simulink library "Weather_Datafile"  (R2018b)
settings: Solver=ode45  StartTime=0.0  StopTime=10.0  RelTol=1e-3  EnableMultiTasking=on
undefined symbols (not defined in the file): DE_TRY2010_04_averageYear, path_carnot
libraries: carnot x1
settings Model: Creator=Bernd.Hafner  LastModifiedBy=P41573
settings DataIOCC: LimitDataPoints=on  SaveFormat=Array  SignalLoggingSaveFormat=ModelDataLogs
settings OptimizationCC: ExpressionDepthLimit=2147483647  LifeSpan=inf
settings DebuggingCC: UnderspecifiedInitializationDetection=Classic  MergeDetectMultiDrivingBlocksExec=none  SolverPrmCheckMsg=warning  FcnCallInpInsideContextMsg=warning  StateNameClashWarn=warning  SFUnexpectedBacktrackingDiag=warning  SFNoUnconditionalDefaultTransitionDiag=warning  SFExecutionAtInitializationDiag=none
settings HardwareCC: ProdBitPerPointer=32  ProdBitPerSizeT=32  ProdBitPerPtrDiffT=32  ProdLargestAtomicFloat=None  ProdIntDivRoundTo=Undefined  ProdEndianess=Unspecified  ProdWordSize=32  ProdHWDeviceType=32-bit Generic
settings ModelReferenceCC: PropagateSignalLabelsOutOfModel=off
settings SFSimCC: SimUseLocalCustomCode=off
settings RTWCC: RTWUseLocalCustomCode=off
settings CodeAppCC: StateflowObjectComments=on
settings GRTTargetCC: TargetLangStandard=C89/C90 (ANSI)  GeneratePreprocessorConditionals=Disable all  CombineOutputUpdateFcns=off  GRTInterface=on
settings ConfigComp: CovMetricSettings=dw  CovHtmlReporting=on  CovSaveCumulativeToWorkspaceVar=on  CovSaveSingleToWorkspaceVar=on  CovExternalEMLEnable=off

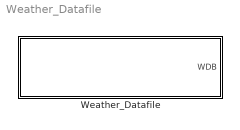
== system Weather_Datafile ==
  Weather_Datafile : Subsystem  mask(Weather Datafile){PathName=path_carnot('data'), FileName='DE_TRY2010_04_averageYear.mat', UserParam=off, VariableName=DE_TRY2010_04_averageYear, SampleTime=3600}
      mask prompts: PathName "Selected path"; FileName "File"; UserParam "Edit file and path"; VariableName "Simulink:blkprm_prompts:FromWksData"; SampleTime "Timestep in data"
      mask help:
      | Loads weather data in a variable in the mask workspace and extends it according to the simulation interval. A "From Workspace" block in the subsystem uses this variable. The file must contain data in the weather data format of Carnot (type "help WDB_format" in Command window). A Unit-Delay with the timestep of the data forces the model to a maximum timestep equal to the data timestep. This "Timestep in data" is shown as information in the "Selection" frame.
      | Use of buttons in the "Picking a file" frame:
      | 1) "From selected path" opens a window to chose a data file from the "Selected path" shown in the "Selection" frame.
      | 2) "Carnot public data" opens a window to chose a data file from the public data folder in Carnot. The "Path" is set to the public data folder.
      | 3) "Carnot internal data" opens a window to chose a data file from the internal data folder in Carnot. The "Path" is set to the internal data folder.
      | "File" shows the name of the selected file, "Path" the folder where it is located. You can allow editing "File" and "Path" with the checkbox. Be aware that the buttons in the "Picking a file" frame will anyway overwrite the edited values.
      mask init:
      | [ok,VariableName] = CarnotCallbacks_Data_from_File('LoadData', ...
      |     gcbh, PathName, FileName);
      mask Help: web(fullfile(path_carnot('help'),'WeatherDatafile.html'),'-helpbrowser')
      mask Callback UserParam: ok = CarnotCallbacks_Data_from_File('UserMaskEnable',gcbh);
      mask TypeOptions VariableName: FromWorkspace/VariableName
      mask TypeOptions SampleTime: UnitDelay/SampleTime
      mask DialogControl ParameterGroupVar Prompt: Picking a file
      mask DialogControl Control2 Prompt: From selected path
      mask DialogControl Control2 Callback: ok = CarnotCallbacks_Data_from_File('GetFilename',gcbh, 'selected');
      mask DialogControl Control3 Prompt: Carnot public data
      mask DialogControl Control3 Callback: ok = CarnotCallbacks_Data_from_File('GetFilename',gcbh, 'public');
      mask DialogControl Control4 Prompt: Carnot internal data
      mask DialogControl Control4 Callback: ok = CarnotCallbacks_Data_from_File('GetFilename',gcbh, 'internal');
      mask DialogControl Container3 Prompt: Chosen file
      mask DialogControl VariableName Prompt: Data:
      mask Display: disp(['Weather data file:\n', FileName(1:end-4)])

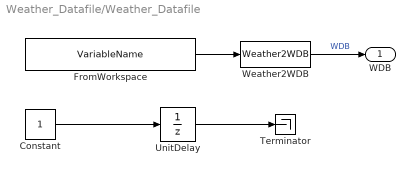
== system Weather_Datafile/Weather_Datafile ==
  Constant : Constant
  FromWorkspace : FromWorkspace  VariableName=VariableName  SampleTime=0  OutputAfterFinalValue=Holding final value
  Terminator : Terminator
  UnitDelay : UnitDelay  SampleTime=SampleTime
  Weather2WDB : carnot/Toolbox/Weather2WDB
      settings: SourceProductName=Carnot
  WDB : Outport
  wires:
  UnitDelay/1 -> Terminator/1
  Constant/1 -> UnitDelay/1
  FromWorkspace/1 -> Weather2WDB/1
  Weather2WDB/1 -> WDB/1  "WDB"
